simulink model "stormAD_Architecture2"  (R2024a)
settings: Solver=FixedStepDiscrete  StartTime=0.0  StopTime=10.0  RelTol=1e-3
model workspace (MAT data in the model file):
  EnvironmentPort = Simulink.Bus
  EnvironmentPort.Alignment = -1
  EnvironmentPort.PreserveElementDimensions = 0
  EnvironmentPort.Elements_internal = Simulink.BusElement
  EnvironmentPort.Elements_internal.DimensionsMode = 'Fixed'
  EnvironmentPort.Elements_internal.SamplingMode = 'Sample based'
  EnvironmentPort.Elements_internal.SampleTime = -1
  EnvironmentPort.Elements_internal.Name = 'fetchEnv'
  EnvironmentPort.Elements_internal.DataType_internal = 'double'
  EnvironmentPort.Elements_internal.Complexity = 'real'
  EnvironmentPort.Elements_internal.Dimensions = 1
  EnvironmentPort.DataScope = 'Auto'
settings Model: Creator=diell  LastModifiedBy=diell

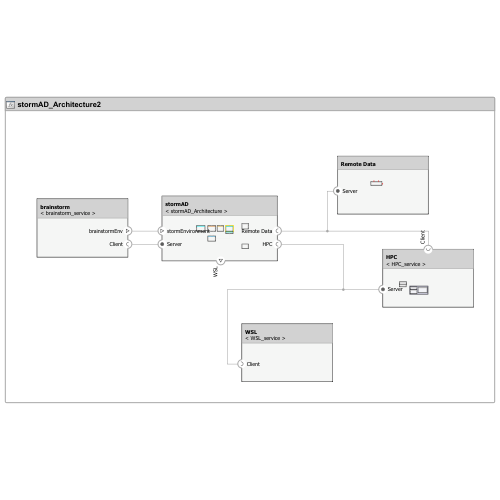
[thumbnail: Simulink's stored preview of the top-level diagram]
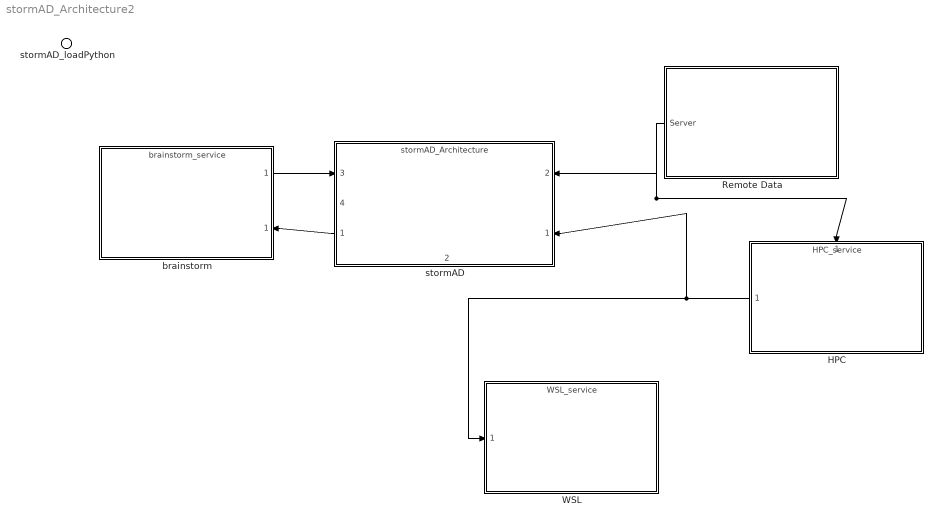
== system stormAD_Architecture2 ==
  stormAD_loadPython : Inport  OutputFunctionCall=on
  HPC : ModelReference  ModelNameDialog=HPC_service  SimulationMode=Normal  ScheduleRates=on  ModelReferenceVersion=1.2
      settings: PortSchema="{\"entries\":[{\"content\":{\"headerSize\":38,\"margin\":15,\"minimumSpacing\":25,\"sides\":[{\"content\":{\"connectorIds\":[\"Out1\"]},\"type\":\"ConnectorPlacement.EquallySpacedRectSide\",\"uuid\":\"7074e736-93ca-48e6-9107-0c0acde2c1e1\"},{\"content\":{\"side\":\"RIGHT\"},\"type\":\"ConnectorPlacement.EquallySpacedRectSide\",\"uuid\":\"49ca3538-4b0a-47e3-9b9f-d0d67086357c\"},{\"content\":{\"connectorIds\":[\"In1\"],\"side\":\"TOP\"},\"type\":\"ConnectorPlacement.EquallySpacedRectSide\",\"uuid\":\"104f6ef2-0cbf-4c6c-8b7e-db8a41d08c3b\"}]},\"type\":\"ConnectorPlacement.EquallySpacedConnector\",\"uuid\":\"4cd04038-0b55-4958-ad0a-aa155b20eca4\"}],\"packageUris\":[\"http://schema.mathworks.com/mf0/Connector/R2020b\"],\"version\":\"1.0\"}"
  Remote Data : Subsystem
      settings: PortSchema="{\"entries\":[{\"content\":{\"headerSize\":26,\"margin\":15,\"minimumSpacing\":25,\"sides\":[{\"content\":{\"connectorIds\":[\"Out1\"]},\"type\":\"ConnectorPlacement.EquallySpacedRectSide\",\"uuid\":\"7074e736-93ca-48e6-9107-0c0acde2c1e1\"},{\"content\":{\"side\":\"RIGHT\"},\"type\":\"ConnectorPlacement.EquallySpacedRectSide\",\"uuid\":\"49ca3538-4b0a-47e3-9b9f-d0d67086357c\"},{\"content\":{\"side\":\"TOP\"},\"type\":\"ConnectorPlacement.EquallySpacedRectSide\",\"uuid\":\"104f6ef2-0cbf-4c6c-8b7e-db8a41d08c3b\"}]},\"type\":\"ConnectorPlacement.EquallySpacedConnector\",\"uuid\":\"4cd04038-0b55-4958-ad0a-aa155b20eca4\"}],\"packageUris\":[\"http://schema.mathworks.com/mf0/Connector/R2020b\"],\"version\":\"1.0\"}"
  WSL : ModelReference  ModelNameDialog=WSL_service  SimulationMode=Normal  ScheduleRates=on  ModelReferenceVersion=1.2
      settings: PortSchema="{\"entries\":[{\"content\":{\"headerSize\":38,\"margin\":15,\"minimumSpacing\":25,\"sides\":[{\"content\":{\"connectorIds\":[\"In1\"]},\"type\":\"ConnectorPlacement.EquallySpacedRectSide\",\"uuid\":\"e4721c40-b49e-4ac5-95ff-3d551931e75b\"},{\"content\":{\"side\":\"RIGHT\"},\"type\":\"ConnectorPlacement.EquallySpacedRectSide\",\"uuid\":\"c82ecebb-3746-4618-8630-b662b5164920\"},{\"content\":{\"side\":\"TOP\"},\"type\":\"ConnectorPlacement.EquallySpacedRectSide\",\"uuid\":\"ab4b1f6e-1a91-4260-a3a9-ab64f2f039dd\"}]},\"type\":\"ConnectorPlacement.EquallySpacedConnector\",\"uuid\":\"1665e1f3-0fa9-43c0-aafb-75b42b6d97af\"}],\"packageUris\":[\"http://schema.mathworks.com/mf0/Connector/R2020b\"],\"version\":\"1.0\"}"
  brainstorm : ModelReference  ModelNameDialog=brainstorm_service  SimulationMode=Normal  ScheduleRates=on  ModelReferenceVersion=1.5
      settings: PortSchema="{\"entries\":[{\"content\":{\"headerSize\":38,\"margin\":15,\"minimumSpacing\":25,\"sides\":[{\"content\":{},\"type\":\"ConnectorPlacement.EquallySpacedRectSide\",\"uuid\":\"e4721c40-b49e-4ac5-95ff-3d551931e75b\"},{\"content\":{\"connectorIds\":[\"Out1\",\"In1\"],\"side\":\"RIGHT\"},\"type\":\"ConnectorPlacement.EquallySpacedRectSide\",\"uuid\":\"c82ecebb-3746-4618-8630-b662b5164920\"},{\"content\":{\"side\":\"TOP\"},\"type\":\"ConnectorPlacement.EquallySpacedRectSide\",\"uuid\":\"ab4b1f6e-1a91-4260-a3a9-ab64f2f039dd\"}]},\"type\":\"ConnectorPlacement.EquallySpacedConnector\",\"uuid\":\"1665e1f3-0fa9-43c0-aafb-75b42b6d97af\"}],\"packageUris\":[\"http://schema.mathworks.com/mf0/Connector/R2020b\"],\"version\":\"1.0\"}"
  stormAD : ModelReference  ModelNameDialog=stormAD_Architecture.slx  SimulationMode=Normal  ScheduleRates=on  ModelReferenceVersion=1.21
      settings: PortSchema="{\"entries\":[{\"content\":{\"headerSize\":38,\"margin\":15,\"minimumSpacing\":25,\"sides\":[{\"content\":{\"connectorIds\":[\"In3\",\"Out1\"]},\"type\":\"ConnectorPlacement.EquallySpacedRectSide\",\"uuid\":\"e4721c40-b49e-4ac5-95ff-3d551931e75b\"},{\"content\":{\"connectorIds\":[\"In2\",\"In1\"],\"side\":\"RIGHT\"},\"type\":\"ConnectorPlacement.EquallySpacedRectSide\",\"uuid\":\"c82ecebb-3746-4618-8630-b662b5164920\"},{\"content\":{\"side\":\"TOP\"},\"type\":\"ConnectorPlacement.EquallySpacedRectSide\",\"uuid\":\"ab4b1f6e-1a91-4260-a3a9-ab64f2f039dd\"},{\"content\":{\"connectorIds\":[\"Out2\"],\"side\":\"BOTTOM\"},\"type\":\"ConnectorPlacement.EquallySpacedRectSide\",\"uuid\":\"af38b5ad-e8e9-44ff-8e82-cc8722ed0521\"},{\"content\":{\"connectorIds\":[\"In4\"],\"side\":\"HIDDEN\"},\"type\":\"ConnectorPlacement.EquallySpacedRectSide\",\"uuid\":\"78c9f743-4b05-4a5f-a08f-1a6cc312c4a0\"}]},\"type\":\"ConnectorPlacement.EquallySpacedConnector\",\"uuid\":\"1665e1f3-0fa9-43c0-aafb-75b42b6d97af\"}],\"packageUris\":[\"http://schema.mathworks.com/mf0/Connector/R2020b\"],\"version\":\"1.0\"}"
  wires:
  stormAD/1 -> brainstorm/1
  HPC/1 -> WSL/1, stormAD/1
  Remote Data/1(Server) -> HPC/1, stormAD/2
  brainstorm/1 -> stormAD/3

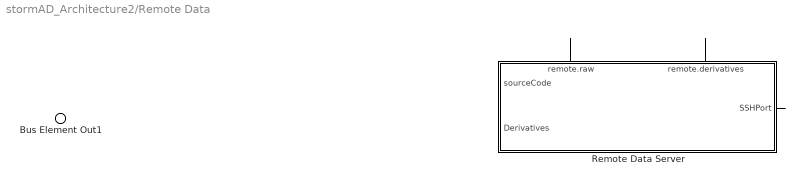
== system stormAD_Architecture2/Remote Data ==
  Remote Data Server : Subsystem
      settings: PortSchema="{\"entries\":[{\"content\":{\"headerSize\":26,\"margin\":15,\"minimumSpacing\":25,\"sides\":[{\"content\":{\"connectorIds\":[\"Out1\",\"In1\"]},\"type\":\"ConnectorPlacement.EquallySpacedRectSide\",\"uuid\":\"d99db108-8c8a-4010-81b2-f142fbf318f5\"},{\"content\":{\"connectorIds\":[\"Out2\"],\"side\":\"RIGHT\"},\"type\":\"ConnectorPlacement.EquallySpacedRectSide\",\"uuid\":\"9190d96c-22e3-4cc9-a507-8f094dc67743\"},{\"content\":{\"connectorIds\":[\"Out3\",\"Out4\"],\"side\":\"TOP\"},\"type\":\"ConnectorPlacement.EquallySpacedRectSide\",\"uuid\":\"08b46875-eac1-4edb-b2eb-5598dd517a75\"},{\"content\":{\"side\":\"BOTTOM\"},\"type\":\"ConnectorPlacement.EquallySpacedRectSide\",\"uuid\":\"000c332a-c8c2-4c2b-a822-ffa253837487\"}]},\"type\":\"ConnectorPlacement.EquallySpacedConnector\",\"uuid\":\"c8d2d02b-cf5a-431f-8876-22d36c8a9b33\"}],\"packageUris\":[\"http://schema.mathworks.com/mf0/Connector/R2020b\"],\"version\":\"1.0\"}"
  Bus Element Out1 : Outport  AllowServiceAccess=on  PortName=Server
  wires:
  Remote Data Server/3(remote.raw) -> ?
  Remote Data Server/4(remote.derivatives) -> ?
  Remote Data Server/2(SSHPort) -> ?

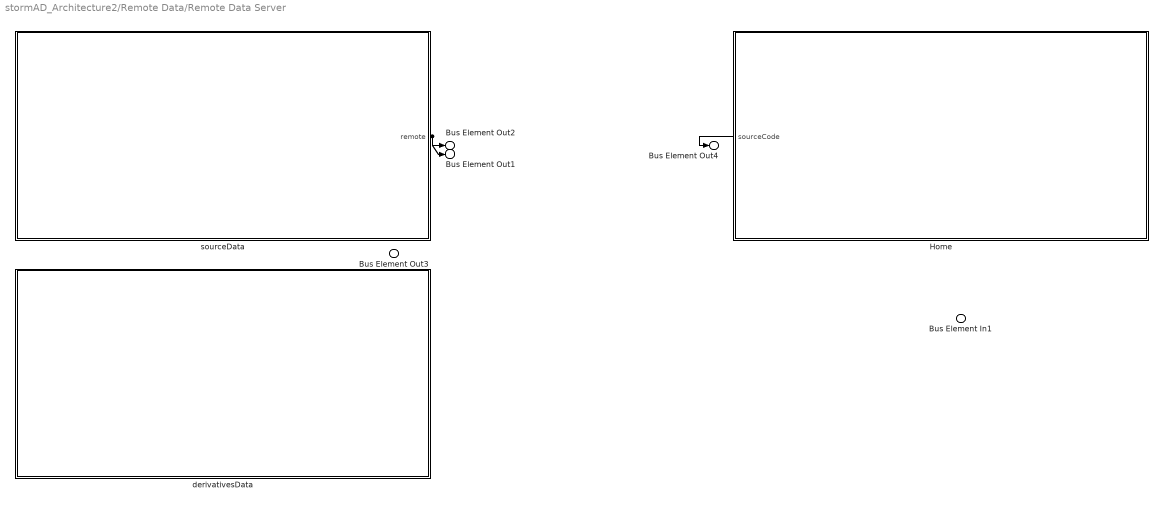
== system stormAD_Architecture2/Remote Data/Remote Data Server ==
  Bus Element In1 : Inport  PortName=Derivatives
  " sourceData" : Subsystem
      settings: PortSchema="{\"entries\":[{\"content\":{\"headerSize\":26,\"margin\":15,\"minimumSpacing\":25,\"sides\":[{\"content\":{},\"type\":\"ConnectorPlacement.EquallySpacedRectSide\",\"uuid\":\"a3539b9a-22db-4da3-b271-35b287ced3a1\"},{\"content\":{\"connectorIds\":[\"Out1\"],\"side\":\"RIGHT\"},\"type\":\"ConnectorPlacement.EquallySpacedRectSide\",\"uuid\":\"72d9f298-5062-46d4-b3c5-f2fa85d7a7a6\"},{\"content\":{\"side\":\"TOP\"},\"type\":\"ConnectorPlacement.EquallySpacedRectSide\",\"uuid\":\"050469fd-3881-4b53-a813-94df038aa659\"}]},\"type\":\"ConnectorPlacement.EquallySpacedConnector\",\"uuid\":\"6db04dad-62f3-4987-a6a9-d236db4fe2a3\"}],\"packageUris\":[\"http://schema.mathworks.com/mf0/Connector/R2020b\"],\"version\":\"1.0\"}"
  Home : Subsystem
      settings: PortSchema="{\"entries\":[{\"content\":{\"headerSize\":26,\"margin\":15,\"minimumSpacing\":25,\"sides\":[{\"content\":{\"connectorIds\":[\"Out1\"]},\"type\":\"ConnectorPlacement.EquallySpacedRectSide\",\"uuid\":\"a3539b9a-22db-4da3-b271-35b287ced3a1\"},{\"content\":{\"side\":\"RIGHT\"},\"type\":\"ConnectorPlacement.EquallySpacedRectSide\",\"uuid\":\"72d9f298-5062-46d4-b3c5-f2fa85d7a7a6\"},{\"content\":{\"side\":\"TOP\"},\"type\":\"ConnectorPlacement.EquallySpacedRectSide\",\"uuid\":\"050469fd-3881-4b53-a813-94df038aa659\"}]},\"type\":\"ConnectorPlacement.EquallySpacedConnector\",\"uuid\":\"6db04dad-62f3-4987-a6a9-d236db4fe2a3\"}],\"packageUris\":[\"http://schema.mathworks.com/mf0/Connector/R2020b\"],\"version\":\"1.0\"}"
  derivativesData : Subsystem
      settings: PortSchema="{\"entries\":[{\"content\":{\"headerSize\":26,\"margin\":15,\"minimumSpacing\":25,\"sides\":[{\"content\":{},\"type\":\"ConnectorPlacement.EquallySpacedRectSide\",\"uuid\":\"a3539b9a-22db-4da3-b271-35b287ced3a1\"},{\"content\":{\"side\":\"RIGHT\"},\"type\":\"ConnectorPlacement.EquallySpacedRectSide\",\"uuid\":\"72d9f298-5062-46d4-b3c5-f2fa85d7a7a6\"},{\"content\":{\"side\":\"TOP\"},\"type\":\"ConnectorPlacement.EquallySpacedRectSide\",\"uuid\":\"050469fd-3881-4b53-a813-94df038aa659\"}]},\"type\":\"ConnectorPlacement.EquallySpacedConnector\",\"uuid\":\"6db04dad-62f3-4987-a6a9-d236db4fe2a3\"}],\"packageUris\":[\"http://schema.mathworks.com/mf0/Connector/R2020b\"],\"version\":\"1.0\"}"
  Bus Element Out4 : Outport  AllowServiceAccess=on  PortName=sourceCode  Element=github
  Bus Element Out3 : Outport  Port=2  AllowServiceAccess=on  PortName=SSHPort
  Bus Element Out1 : Outport  Port=3  AllowServiceAccess=on  PortName=remote.raw
  Bus Element Out2 : Outport  Port=4  AllowServiceAccess=on  PortName=remote.derivatives
  wires:
  " sourceData"/1(remote) -> Bus Element Out1/1, Bus Element Out2/1
  Home/1(sourceCode) -> Bus Element Out4/1

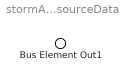
== system stormAD_Architecture2/Remote Data/Remote Data Server/ sourceData ==
  Bus Element Out1 : Outport  AllowServiceAccess=on  PortName=remote

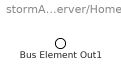
== system stormAD_Architecture2/Remote Data/Remote Data Server/Home ==
  Bus Element Out1 : Outport  AllowServiceAccess=on  PortName=sourceCode

== system stormAD_Architecture2/Remote Data/Remote Data Server/derivativesData ==
